simulink model "Kirk_Phase3"  (R2020a)
settings: Solver=FixedStepAuto  StartTime=0.0  StopTime=tsim  FixedStep=baseRate  RelTol=1e-3  EnableMultiTasking=on
values from neighbouring files (symbols this model uses):
  a1 = str2double(environment_file(search_start(1)+length(value)+1:search_start(1)+search_end(1)-2))    [Run_Initializer.m]
  a2 = str2double(environment_file(search_start(1)+length(value)+1:search_start(1)+search_end(1)-2))    [Run_Initializer.m]
  a3 = str2double(environment_file(search_start(1)+length(value)+1:search_start(1)+search_end(1)-2))    [Run_Initializer.m]
  b0 = str2double(environment_file(search_start(1)+length(value)+1:search_start(1)+search_end(1)-2))    [Run_Initializer.m]
  b1 = str2double(environment_file(search_start(1)+length(value)+1:search_start(1)+search_end(1)-2))    [Run_Initializer.m]
  b2 = str2double(environment_file(search_start(1)+length(value)+1:search_start(1)+search_end(1)-2))    [Run_Initializer.m]
  baseRate = 1/20    (= 0.05)    [Run_Initializer.m]
  bring_arm_to_rest_time = 3    [Run_Initializer.m]
  drop_states_BLACK = [ 2.33; 1.2; target_starting_angle]    [Run_Initializer.m]
  drop_states_BLUE = [ xLength/2+0.9; yLength/2+0.5; 0]    [Run_Initializer.m]
  drop_states_RED = [ 1.16; 1.2; 0]    [Run_Initializer.m]
  elbow_max_omega = 30*pi/180    (= 0.523598775598)    [Run_Initializer.m]
  F_thrusters_BLACK = 0.25.*ones(8,1)    [Run_Initializer.m]
  F_thrusters_BLUE = 0.25.*ones(8,1)    [Run_Initializer.m]
  F_thrusters_RED = 0.25.*ones(8,1)    [Run_Initializer.m]
  home_states_BLACK = [ 2.33; 1.2; target_starting_angle]    [Run_Initializer.m]
  home_states_BLUE = [ xLength/2-0.9; yLength/2+0.5; 0]    [Run_Initializer.m]
  home_states_RED = [ 1.16; 1.2; 0]    [Run_Initializer.m]
  I0 = str2double(environment_file(search_start(1)+length(value)+1:search_start(1)+search_end(1)-2))    [Run_Initializer.m]
  I1 = str2double(environment_file(search_start(1)+length(value)+1:search_start(1)+search_end(1)-2))    [Run_Initializer.m]
  I2 = str2double(environment_file(search_start(1)+length(value)+1:search_start(1)+search_end(1)-2))    [Run_Initializer.m]
  I3 = str2double(environment_file(search_start(1)+length(value)+1:search_start(1)+search_end(1)-2))    [Run_Initializer.m]
  init_states_BLACK = [ 2.33; 1.2; target_starting_angle]    [Run_Initializer.m]
  init_states_BLUE = [ xLength/2+0.9; yLength/2+0.5; 0]    [Run_Initializer.m]
  init_states_RED = [ 1.16; 1.2; 0]    [Run_Initializer.m]
  joint_limit_buffer_angle = 0    [Run_Initializer.m]
  Kd_tb = 0.4/5    (= 0.08)    [Run_Initializer.m]
  Kd_tblue = 0.4    [Run_Initializer.m]
  Kd_tr = 0.4    [Run_Initializer.m]
  Kd_xb = 5    [Run_Initializer.m]
  Kd_xblue = 5    [Run_Initializer.m]
  Kd_xr = 5    [Run_Initializer.m]
  Kd_yb = 5    [Run_Initializer.m]
  Kd_yblue = 5    [Run_Initializer.m]
  Kd_yr = 5    [Run_Initializer.m]
  KI_vel_PI = 0    [Run_Initializer.m]
  KI_vel_PI_theta = 0    [Run_Initializer.m]
  Kp_tb = 0.1/5    (= 0.02)    [Run_Initializer.m]
  Kp_tblue = 0.1    [Run_Initializer.m]
  Kp_tr = 0.1    [Run_Initializer.m]
  Kp_vel_PI = 40    [Run_Initializer.m]
  Kp_vel_PI_theta = 0.6    [Run_Initializer.m]
  Kp_xb = 2    [Run_Initializer.m]
  Kp_xblue = 2    [Run_Initializer.m]
  Kp_xr = 2    [Run_Initializer.m]
  Kp_yb = 2    [Run_Initializer.m]
  Kp_yblue = 2    [Run_Initializer.m]
  Kp_yr = 2    [Run_Initializer.m]
  m0 = str2double(environment_file(search_start(1)+length(value)+1:search_start(1)+search_end(1)-2))    [Run_Initializer.m]
  m1 = str2double(environment_file(search_start(1)+length(value)+1:search_start(1)+search_end(1)-2))    [Run_Initializer.m]
  m2 = str2double(environment_file(search_start(1)+length(value)+1:search_start(1)+search_end(1)-2))    [Run_Initializer.m]
  m3 = str2double(environment_file(search_start(1)+length(value)+1:search_start(1)+search_end(1)-2))    [Run_Initializer.m]
  max_body_omega = 15*pi/180    (= 0.261799387799)    [Run_Initializer.m]
  max_x_velocity = 0.1    [Run_Initializer.m]
  max_y_velocity = 0.1    [Run_Initializer.m]
  noise_variance_BLACK = 0    [Run_Initializer.m]
  noise_variance_BLUE = 0    [Run_Initializer.m]
  noise_variance_RED = 0    [Run_Initializer.m]
  Phase0_End = Phase0_Duration    (= 5)    [Run_Initializer.m]
  Phase1_End = Phase0_Duration + Phase1_Duration    (= 10)    [Run_Initializer.m]
  Phase2_End = Phase0_Duration + Phase1_Duration +                                   Phase2_Duration    (= 35)    [Run_Initializer.m]
  Phase3_End = Phase0_Duration + Phase1_Duration +                                   Phase2_Duration + Phase3_Duration    (= 95)    [Run_Initializer.m]
  Phase3_SubPhase1_End = Phase2_End + Phase3_SubPhase1_Duration    (= 35)    [Run_Initializer.m]
  Phase3_SubPhase2_End = Phase2_End + Phase3_SubPhase1_Duration +                                   Phase3_SubPhase2_Duration    (= 35)    [Run_Initializer.m]
  Phase3_SubPhase3_End = Phase2_End + Phase3_SubPhase1_Duration +                                   Phase3_SubPhase2_Duration +                                  Phase3_SubPhase3_Duration    (= 35)    [Run_Initializer.m]
  Phase3_SubPhase4_End = Phase2_End + Phase3_SubPhase1_Duration +                                   Phase3_SubPhase2_Duration +                                  Phase3_SubPhase3_Duration +                                  Phase3_SubPhase4_Duration    [Run_Initializer.m]
  Phase4_End = Phase0_Duration + Phase1_Duration +                                   Phase2_Duration + Phase3_Duration +                                   Phase4_Duration    (= 115)    [Run_Initializer.m]
  Phase5_End = Phase0_Duration + Phase1_Duration +                                   Phase2_Duration + Phase3_Duration +                                   Phase4_Duration + Phase5_Duration    (= 120)    [Run_Initializer.m]
  phi = str2num(erase(environment_file(search_start(1)+length(value)+1:search_start(1)+search_end(1)-2),'np.'))    [Run_Initializer.m]
  serverRate = 1/10    (= 0.1)    [Run_Initializer.m]
  shoulder_max_omega = 30*pi/180    (= 0.523598775598)    [Run_Initializer.m]
  target_angular_velocity = 0.    (= 0)    [Run_Initializer.m]
  thruster_dist2CG_BLACK = [83.42;-52.58;55.94;-60.05;54.08;-53.92;77.06;-55.94]    [Run_Initializer.m]
  thruster_dist2CG_BLUE = [83.42;-52.58;55.94;-60.05;54.08;-53.92;77.06;-55.94]    [Run_Initializer.m]
  thruster_dist2CG_RED = [49.92;-78.08;70.46;-63.54;81.08;-50.42;57.44;-75.96]    [Run_Initializer.m]
  wrist_max_omega = 30*pi/180    (= 0.523598775598)    [Run_Initializer.m]
undefined symbols (not defined in the file or in its folder): DiscIntNeverNeededParam, platformSelection, simMode, WhoAmI
libraries: dspstat3 x18, dspsigops x12, raspberrypiBasiclib x10, MainLibrary x10, embdlinuxlib x8, simulink x8, mspfiltlib x3, dsparch4 x3, dspswit3 x2, sensehatlib x1
(part 12 of 12)

== matlab function Kirk_Phase3/Phase #3: Experiment/Change RED Behavior/Sub-Phase #4/Custom Integral Acceleration Controller1/Sample and Hold Data to Match PhaseSpace (RED)/MATLAB Function ==
  data: TIME input; y output; SERVER input
function y = fcn(TIME, SERVER)

if mod(TIME,SERVER) == 0
    y = 1;
else
    y = 0;
end

== matlab function Kirk_Phase3/Phase #3: Experiment/Change RED Behavior/Sub-Phase #4/Custom Integral Acceleration Controller2/Sample and Hold Data to Match PhaseSpace (RED)/MATLAB Function ==
  data: TIME input; y output; SERVER input
function y = fcn(TIME, SERVER)

if mod(TIME,SERVER) == 0
    y = 1;
else
    y = 0;
end

== matlab function Kirk_Phase3/Phase #3: Experiment/Change BLACK Behavior/Sub-Phase #2 /Hough Control/MATLAB Function2 ==
  data: Oy output; z input; Ox output
function [Oy, Ox]   = C3( z )
%C3 gives the rotation matrix about the z-axis for an angle 'z'
%   z - the angle about the z-axis which you rotate
%   A - the rotation matrix

Ox = [cos(z) sin(z); -sin(z) cos(z)]*[1;0];
Oy = [cos(z) sin(z); -sin(z) cos(z)]*[0;1];
end

== matlab function Kirk_Phase3/Phase #3: Experiment/Change BLACK Behavior/Sub-Phase #2 /Hough Control/MATLAB Function3 ==
  data: z input; Ox output
function Ox    = C3( z )
%C3 gives the rotation matrix about the z-axis for an angle 'z'
%   z - the angle about the z-axis which you rotate
%   A - the rotation matrix

Ox = [cos(z) sin(z); -sin(z) cos(z)]*[1;0];
end

== matlab function Kirk_Phase3/Phase #3: Experiment/Change BLACK Behavior/Sub-Phase #2 /Hough Control/MATLAB Function4 ==
  data: Oy input; e_out output; e_in input
function e_out = fcn(Oy, e_in)

a = sign(Oy'*e_in);
e_out = -a*norm(e_in);

== matlab function Kirk_Phase3/Phase #3: Experiment/Change BLACK Behavior/Sub-Phase #3 /Hough Control/MATLAB Function2 ==
  data: Oy output; z input; Ox output
function [Oy, Ox]   = C3( z )
%C3 gives the rotation matrix about the z-axis for an angle 'z'
%   z - the angle about the z-axis which you rotate
%   A - the rotation matrix

Ox = [cos(z) sin(z); -sin(z) cos(z)]*[1;0];
Oy = [cos(z) sin(z); -sin(z) cos(z)]*[0;1];
end

== matlab function Kirk_Phase3/From Force//Torque to PWM Signal/Change BLUE Behavior/Calculate Thruster ON//OFF/MATLAB Function ==
  data: H output; thruster_dist2CG_BLUE parameter; F_thrusters_BLUE parameter
function H = MakeH(thruster_dist2CG_BLUE,F_thrusters_BLUE)

Vec1 = [ -1
         -1
          0 
          0
          1
          1
          0
          0 ];
      
Vec2 = [  0
          0
          1
          1
          0
          0
         -1
         -1 ];
     
Vec3 = thruster_dist2CG_BLUE./1000;

Mat1 = [Vec1, Vec2, Vec3]';

Mat2 = diag((F_thrusters_BLUE./2));

H    = Mat1*Mat2;

end

== matlab function Kirk_Phase3/Phase #3: Experiment/Change BLACK Behavior/Sub-Phase #3 /Hough Control/MATLAB Function3 ==
  data: z input; Ox output
function Ox    = C3( z )
%C3 gives the rotation matrix about the z-axis for an angle 'z'
%   z - the angle about the z-axis which you rotate
%   A - the rotation matrix

Ox = [cos(z) sin(z); -sin(z) cos(z)]*[1;0];
end

== matlab function Kirk_Phase3/Phase #3: Experiment/Change BLACK Behavior/Sub-Phase #3 /Hough Control/MATLAB Function4 ==
  data: Oy input; e_out output; e_in input
function e_out = fcn(Oy, e_in)

a = sign(Oy'*e_in);
e_out = -a*norm(e_in);

== matlab function Kirk_Phase3/Phase #3: Experiment/Change RED Behavior/Sub-Phase #4/wind down upon capture ==
  data: omega1_in input; omega2_in input; omega3_in input; omega1_out output; is_target_captured input; omega2_out output; omega3_out output; serverRate parameter; bring_arm_to_rest_time parameter; accel_time_ms output
function [omega1_out, omega2_out, omega3_out, accel_time_ms] = are_we_winding_down(omega1_in, omega2_in, omega3_in, is_target_captured, serverRate, bring_arm_to_rest_time)

if is_target_captured
    omega1_out = 0;
    omega2_out = 0;
    omega3_out = 0;
    accel_time_ms = bring_arm_to_rest_time*1000;
else
    omega1_out = omega1_in;
    omega2_out = omega2_in;
    omega3_out = omega3_in;
    accel_time_ms = serverRate*1000;
end

== matlab function Kirk_Phase3/Phase #3: Experiment/Change RED Behavior/Sub-Phase #4/wind down upon_capture2 ==
  data: Fx_in input; Fy_in input; Tz_in input; Fx_out output; is_target_captured input; Fy_out output; Tz_out output
function [Fx_out, Fy_out, Tz_out] = are_we_winding_down(Fx_in, Fy_in, Tz_in, is_target_captured)

if is_target_captured
    Fx_out = 0;
    Fy_out = 0;
    Tz_out = 0;
else
    Fx_out = Fx_in;
    Fy_out = Fy_in;
    Tz_out = Tz_in;
end

== matlab function Kirk_Phase3/Phase #3: Experiment/Change RED Behavior/Sub-Phase #4/calculate_mass_matrix ==
  data: q0_d input; M output; q1_d input; q2_d input; q3_d input; I0 parameter; I1 parameter; I2 parameter; I3 parameter; a1 parameter; a2 parameter; a3 parameter; b0 parameter; b1 parameter; b2 parameter; m0 parameter; m1 parameter; m2 parameter; m3 parameter; phi parameter
function M  = generate_M(q0_d,q1_d,q2_d,q3_d,I0, I1, I2, I3, a1, a2, a3, b0, b1, b2, m0, m1, m2, m3, phi)

t2 = a1+b1;
t3 = a1.*m1;
t4 = m2.*t2;
t5 = m3.*t2;
t6 = q0_d+q1_d;
t7 = cos(t6);
t8 = t3+t4+t5;           
t9 = a2.*m2;
t10 = a2+b2;
t11 = m3.*t10;
t12 = q0_d+q1_d+q2_d;
t13 = cos(t12);
t14 = t9+t11;
t15 = q0_d+q1_d+q2_d+q3_d;
t16 = cos(t15);
t17 = m0+m1+m2+m3;
t18 = b0.*m1;
t19 = b0.*m2;
t20 = b0.*m3;
t21 = t18+t19+t20;
t22 = phi+q0_d;
t23 = sin(t6);
t24 = sin(t12);
t25 = sin(t15);
t26 = a2.*m3;
t27 = b2.*m3;
t28 = t9+t26+t27;
t29 = sin(t22);
t86 = t7.*t8;
t87 = t13.*t14;
t88 = a3.*m3.*t16;
t30 = -t86-t87-t88-t21.*t29;
t31 = cos(t22);
t32 = t21.*t31;
t89 = t8.*t23;
t90 = t14.*t24;
t91 = a3.*m3.*t25;
t33 = t32-t89-t90-t91;
t34 = a1.^2;
t35 = a2.^2;
t36 = b0.^2;
t37 = b1.^2;
t38 = a1.*a2.*m2.*2.0;
t39 = a1.*a2.*m3.*2.0;
t40 = a2.*b1.*m2.*2.0;
t41 = a1.*b2.*m3.*2.0;
t42 = a2.*b1.*m3.*2.0;
t43 = b1.*b2.*m3.*2.0;
t44 = t38+t39+t40+t41+t42+t43;
t45 = cos(q2_d);
t46 = t44.*t45;
t47 = a2.*a3.*m3.*2.0;
t48 = a3.*b2.*m3.*2.0;
t49 = t47+t48;
t50 = cos(q3_d);
t51 = t49.*t50;
t52 = a1.*a3.*m3.*2.0;
t53 = a3.*b1.*m3.*2.0;
t54 = t52+t53;
t55 = q2_d+q3_d;
t56 = cos(t55);
t57 = t54.*t56;
t58 = phi-q1_d;
t59 = sin(t58);
t60 = -phi+q1_d+q2_d;
t61 = sin(t60);
t62 = -phi+q1_d+q2_d+q3_d;
t63 = sin(t62);
t64 = m1.*t34;
t65 = m2.*t34;
t66 = m3.*t34;
t67 = m2.*t35;
t68 = m3.*t35;
t69 = a3.^2;
t70 = m3.*t69;
t71 = m2.*t37;
t72 = m3.*t37;
t73 = b2.^2;
t74 = m3.*t73;
t75 = a1.*b1.*m2.*2.0;
t76 = a1.*b1.*m3.*2.0;
t77 = a2.*b2.*m3.*2.0;
t78 = a2.*b0.*m2;
t79 = a2.*b0.*m3;
t80 = b0.*b2.*m3;
t81 = t78+t79+t80;
t82 = a1.*a3.*m3;
t83 = a3.*b1.*m3;
t84 = t82+t83;
t85 = t56.*t84;
t92 = a1.*b0.*m1;
t93 = a1.*b0.*m2;
t94 = a1.*b0.*m3;
t95 = b0.*b1.*m2;
t96 = b0.*b1.*m3;
t97 = t92+t93+t94+t95+t96;
t98 = t59.*t97;
t112 = t61.*t81;
t113 = a3.*b0.*m3.*t63;
t99 = I1+I2+I3+t46+t51+t57+t64+t65+t66+t67+t68+t70+t71+t72+t74+t75+t76+t77+t98-t112-t113;
t100 = a1.*a2.*m2;
t101 = a1.*a2.*m3;
t102 = a2.*b1.*m2;
t103 = a1.*b2.*m3;
t104 = a2.*b1.*m3;
t105 = b1.*b2.*m3;
t106 = t100+t101+t102+t103+t104+t105;
t107 = t45.*t106;
t108 = a2.*a3.*m3;
t109 = a3.*b2.*m3;
t110 = t108+t109;
t111 = t50.*t110;
t114 = I2+I3+t51+t67+t68+t70+t74+t77+t85+t107;
t115 = I3+t70+t85+t111;
t116 = I3+t70+t111;
M = reshape([t17,0.0,t30,-t86-t87-t88,-t88-t13.*t28,-t88,0.0,t17,t33,-t89-t90-t91,-t91-t24.*t28,-t91,t30,t33,I0+I1+I2+I3+t46+t51+t57+t64+t65+t66+t67+t68+t70+t71+t72+t74+t75+t76+t77+t59.*(a1.*b0.*m1.*2.0+a1.*b0.*m2.*2.0+a1.*b0.*m3.*2.0+b0.*b1.*m2.*2.0+b0.*b1.*m3.*2.0)+m1.*t36+m2.*t36+m3.*t36-t61.*(a2.*b0.*m2.*2.0+a2.*b0.*m3.*2.0+b0.*b2.*m3.*2.0)-a3.*b0.*m3.*t63.*2.0,t99,I2+I3+t51+t67+t68+t70+t74+t77+t85+t107-t112-t113,I3+t70+t85+t111-t113,-t7.*t8-t13.*t14-a3.*m3.*t16,-t8.*t23-t14.*t24-a3.*m3.*t25,t99,I1+I2+I3+t46+t51+t57+t64+t65+t66+t67+t68+t70+t71+t72+t74+t75+t76+t77,t114,t115,-t13.*t28-a3.*m3.*t16,-t24.*t28-a3.*m3.*t25,I2+I3+t51+t67+t68+t70+t74+t77+t85+t107-t61.*t81-a3.*b0.*m3.*t63,t114,I2+I3+t51+t67+t68+t70+t74+t77,t116,-a3.*m3.*t16,-a3.*m3.*t25,I3+t70+t85+t111-a3.*b0.*m3.*t63,t115,t116,I3+t70],[6,6]);

== matlab function Kirk_Phase3/Phase #3: Experiment/Change RED Behavior/Sub-Phase #4/calculate_coriolis_matrix ==
  data: q0_d input; C output; q1_d input; q2_d input; q3_d input; q0_dot_d input; q1_dot_d input; q2_dot_d input; q3_dot_d input; a1 parameter; a2 parameter; a3 parameter; b0 parameter; b1 parameter; b2 parameter; m1 parameter; m2 parameter; m3 parameter; phi parameter
function C  = generate_C(q0_d,q1_d,q2_d,q3_d, q0_dot_d,q1_dot_d,q2_dot_d,q3_dot_d, a1, a2, a3, b0, b1, b2, m1, m2, m3, phi)

t2 = a1+b1;
t3 = a1.*m1;
t4 = m2.*t2;
t5 = m3.*t2;
t6 = t3+t4+t5;
t7 = a2.*m2;
t8 = a2+b2;
t9 = m3.*t8;
t10 = t7+t9;
t11 = pi.*(1.0./2.0);
t12 = q0_dot_d.*t6;
t13 = q1_dot_d.*t6;
t14 = q0_d+q1_d+t11;
t15 = cos(t14);
t16 = t12+t13;
t17 = q0_dot_d.*t10;
t18 = q1_dot_d.*t10;
t19 = q2_dot_d.*t10;
t20 = q0_d+q1_d+q2_d+t11;
t21 = cos(t20);
t22 = t17+t18+t19;
t23 = a3.*m3.*q0_dot_d;
t24 = a3.*m3.*q1_dot_d;
t25 = a3.*m3.*q2_dot_d;
t26 = a3.*m3.*q3_dot_d;
t27 = q0_d+q1_d+q2_d+q3_d+t11;
t28 = cos(t27);
t29 = t23+t24+t25+t26;
t30 = b0.*m1;
t31 = b0.*m2;
t32 = b0.*m3;
t33 = t30+t31+t32;
t34 = phi+q0_d;
t35 = sin(t14);
t36 = sin(t20);
t37 = sin(t27);
t38 = q0_dot_d+q1_dot_d+q2_dot_d+q3_dot_d;
t39 = q0_d+q1_d+q2_d+q3_d;
t40 = a1.*b0.*m1.*q1_dot_d;
t41 = a1.*b0.*m2.*q1_dot_d;
t42 = a1.*b0.*m3.*q1_dot_d;
t43 = b0.*b1.*m2.*q1_dot_d;
t44 = b0.*b1.*m3.*q1_dot_d;
t45 = phi-q1_d;
t46 = cos(t45);
t47 = a2.*b0.*m2.*q1_dot_d;
t48 = a2.*b0.*m2.*q2_dot_d;
t49 = a2.*b0.*m3.*q1_dot_d;
t50 = a2.*b0.*m3.*q2_dot_d;
t51 = b0.*b2.*m3.*q1_dot_d;
t52 = b0.*b2.*m3.*q2_dot_d;
t53 = -phi+q1_d+q2_d;
t54 = cos(t53);
t55 = a3.*b0.*m3.*q1_dot_d;
t56 = a3.*b0.*m3.*q2_dot_d;
t57 = a3.*b0.*m3.*q3_dot_d;
t58 = -phi+q1_d+q2_d+q3_d;
t59 = cos(t58);
t60 = a2.*b1.*m2.*q2_dot_d;
t61 = a1.*b2.*m3.*q2_dot_d;
t62 = a2.*b1.*m3.*q2_dot_d;
t63 = b1.*b2.*m3.*q2_dot_d;
t64 = a1.*a2.*m2.*q2_dot_d;
t65 = a1.*a2.*m3.*q2_dot_d;
t66 = sin(q2_d);
t67 = t60+t61+t62+t63+t64+t65;
t68 = a3.*b2.*m3.*q3_dot_d;
t69 = a2.*a3.*m3.*q3_dot_d;
t70 = sin(q3_d);
t71 = t68+t69;
t72 = a3.*b1.*m3.*q2_dot_d;
t73 = a3.*b1.*m3.*q3_dot_d;
t74 = a1.*a3.*m3.*q2_dot_d;
t75 = a1.*a3.*m3.*q3_dot_d;
t76 = q2_d+q3_d;
t77 = sin(t76);
t78 = t72+t73+t74+t75;
t79 = a2.*b0.*m2.*q0_dot_d;
t80 = a2.*b0.*m3.*q0_dot_d;
t81 = b0.*b2.*m3.*q0_dot_d;
t82 = t47+t48+t49+t50+t51+t52+t79+t80+t81;
t83 = a3.*b0.*m3.*q0_dot_d;
t84 = t55+t56+t57+t83;
t85 = a1.*b0.*m1.*q0_dot_d;
t86 = a1.*b0.*m2.*q0_dot_d;
t87 = a1.*b0.*m3.*q0_dot_d;
t88 = b0.*b1.*m2.*q0_dot_d;
t89 = b0.*b1.*m3.*q0_dot_d;
t90 = a2.*b1.*m2.*q0_dot_d;
t91 = a1.*b2.*m3.*q0_dot_d;
t92 = a2.*b1.*m2.*q1_dot_d;
t93 = a2.*b1.*m3.*q0_dot_d;
t94 = a1.*b2.*m3.*q1_dot_d;
t95 = a2.*b1.*m3.*q1_dot_d;
t96 = b1.*b2.*m3.*q0_dot_d;
t97 = b1.*b2.*m3.*q1_dot_d;
t98 = a1.*a2.*m2.*q0_dot_d;
t99 = a1.*a2.*m2.*q1_dot_d;
t100 = a1.*a2.*m3.*q0_dot_d;
t101 = a1.*a2.*m3.*q1_dot_d;
t102 = t60+t61+t62+t63+t64+t65+t90+t91+t92+t93+t94+t95+t96+t97+t98+t99+t100+t101;
t103 = a3.*b1.*m3.*q0_dot_d;
t104 = a3.*b1.*m3.*q1_dot_d;
t105 = a1.*a3.*m3.*q0_dot_d;
t106 = a1.*a3.*m3.*q1_dot_d;
t107 = t72+t73+t74+t75+t103+t104+t105+t106;
t108 = t79+t80+t81;
t109 = t54.*t108;
t110 = t59.*t83;
t111 = t90+t91+t92+t93+t94+t95+t96+t97+t98+t99+t100+t101;
t112 = t66.*t111;
t113 = t103+t104+t105+t106;
t114 = t77.*t113;
t115 = a2.*q0_dot_d;
t116 = a2.*q1_dot_d;
t117 = a2.*q2_dot_d;
t118 = b2.*q0_dot_d;
t119 = b2.*q1_dot_d;
t120 = b2.*q2_dot_d;
t121 = t115+t116+t117+t118+t119+t120;
t122 = a3.*m3.*t70.*t121;
t123 = a1.*q0_dot_d;
t124 = a1.*q1_dot_d;
t125 = b1.*q0_dot_d;
t126 = b1.*q1_dot_d;
t127 = t123+t124+t125+t126;
t128 = a3.*m3.*t77.*t127;
C = reshape([0.0,0.0,0.0,0.0,0.0,0.0,0.0,0.0,0.0,0.0,0.0,0.0,-t15.*t16-t21.*t22-t28.*t29-q0_dot_d.*t33.*cos(t34),-t16.*t35-t22.*t36-t29.*t37-q0_dot_d.*t33.*sin(t34),-t66.*t67-t70.*t71-t77.*t78-t46.*(t40+t41+t42+t43+t44)-t59.*(t55+t56+t57)-t54.*(t47+t48+t49+t50+t51+t52),t109+t110-t66.*t67-t70.*t71-t77.*t78+t46.*(t85+t86+t87+t88+t89),t109+t110+t112+t114-t70.*t71,t110+t122+t128,-t15.*t16-t21.*t22-t28.*t29,-t16.*t35-t22.*t36-t29.*t37,-t66.*t67-t54.*t82-t70.*t71-t59.*t84-t77.*t78-t46.*(t40+t41+t42+t43+t44+t85+t86+t87+t88+t89),-t66.*t67-t70.*t71-t77.*t78,t112+t114-t70.*t71,t122+t128,-t21.*t22-t28.*t29,-t22.*t36-t29.*t37,-t54.*t82-t70.*t71-t59.*t84-t66.*t102-t77.*t107,-t70.*t71-t66.*t102-t77.*t107,-a3.*m3.*q3_dot_d.*t8.*t70,a3.*m3.*t8.*t70.*(q0_dot_d+q1_dot_d+q2_dot_d),a3.*m3.*t38.*sin(t39),-a3.*m3.*t38.*cos(t39),-a3.*b0.*m3.*t38.*t59-a3.*m3.*t8.*t38.*t70-a3.*m3.*t2.*t38.*t77,-a3.*m3.*t8.*t38.*t70-a3.*m3.*t2.*t38.*t77,-a3.*m3.*t8.*t38.*t70,0.0],[6,6]);

== matlab function Kirk_Phase3/From Force//Torque to PWM Signal/Change BLUE Behavior/Calculate Thruster ON//OFF/MATLAB Function1 ==
  data: H output; thruster_dist2CG_BLUE parameter; F_thrusters_BLUE parameter
function H = MakeH(thruster_dist2CG_BLUE,F_thrusters_BLUE)

Vec1 = [ -1
         -1
          0 
          0
          1
          1
          0
          0 ];
      
Vec2 = [  0
          0
          1
          1
          0
          0
         -1
         -1 ];
     
Vec3 = thruster_dist2CG_BLUE./1000;

Mat1 = [Vec1, Vec2, Vec3]';

Mat2 = diag((F_thrusters_BLUE./2));

H    = Mat1*Mat2;

end

== matlab function Kirk_Phase3/From Force//Torque to PWM Signal/Change RED Behavior/Calculate Thruster ON//OFF/MATLAB Function3 ==
  data: H output; thruster_dist2CG_RED parameter; F_thrusters_RED parameter
function H = MakeH(thruster_dist2CG_RED,F_thrusters_RED)

Vec1 = [ -1
         -1
          0 
          0
          1
          1
          0
          0 ];
      
Vec2 = [  0
          0
          1
          1
          0
          0
         -1
         -1 ];
     
Vec3 = thruster_dist2CG_RED./1000;

Mat1 = [Vec1, Vec2, Vec3]';

Mat2 = diag((F_thrusters_RED./2));

H    = Mat1*Mat2;

end

== matlab function Kirk_Phase3/From Force//Torque to PWM Signal/Change RED Behavior/Calculate Thruster ON//OFF/MATLAB Function4 ==
  data: H output; thruster_dist2CG_RED parameter; F_thrusters_RED parameter; theta_1 input; theta_2 input; theta_3 input; b0 parameter; phi parameter; a1 parameter; b1 parameter; a2 parameter; b2 parameter; a3 parameter; m0 parameter; m1 parameter; m2 parameter; m3 parameter
function H = MakeH(thruster_dist2CG_RED,F_thrusters_RED, theta_1, theta_2, theta_3, b0, phi, a1, b1, a2, b2, a3,m0, m1, m2, m3)

link1_com_x = b0*cos(phi) + a1*cos(pi/2 + theta_1);
link1_com_y = b0*sin(phi) + a1*sin(pi/2 + theta_1);

link2_com_x = link1_com_x + b1*cos(pi/2 + theta_1) + a2*cos(pi/2 + theta_1 + theta_2);
link2_com_y = link1_com_y + b1*sin(pi/2 + theta_1) + a2*sin(pi/2 + theta_1 + theta_2);

link3_com_x = link2_com_x + b2*cos(pi/2 + theta_1 + theta_2) + a3*cos(pi/2 + theta_1 + theta_2 + theta_3);
link3_com_y = link2_com_y + b2*sin(pi/2 + theta_1 + theta_2) + a3*sin(pi/2 + theta_1 + theta_2 + theta_3);

delta_com_due_to_arm_x = (m1*link1_com_x + m2*link2_com_x + m3*link3_com_x)/(m0 + m1 + m2 + m3)*1000; % [mm]
delta_com_due_to_arm_y = (m1*link1_com_y + m2*link2_com_y + m3*link3_com_y)/(m0 + m1 + m2 + m3)*1000; % [mm]

adjusted_thruster_dist2CG_RED = [thruster_dist2CG_RED(1)-delta_com_due_to_arm_y;
                                 thruster_dist2CG_RED(2)-delta_com_due_to_arm_y;
                                 thruster_dist2CG_RED(3)-delta_com_due_to_arm_x;
                                 thruster_dist2CG_RED(4)-delta_com_due_to_arm_x;
                                 thruster_dist2CG_RED(5)+delta_com_due_to_arm_y;
                                 thruster_dist2CG_RED(6)+delta_com_due_to_arm_y;
                                 thruster_dist2CG_RED(7)+delta_com_due_to_arm_x;
                                 thruster_dist2CG_RED(8)+delta_com_due_to_arm_x];
                                 


Vec1 = [ -1
         -1
          0 
          0
          1
          1
          0
          0 ];
      
Vec2 = [  0
          0
          1
          1
          0
          0
         -1
         -1 ];
     
Vec3 = adjusted_thruster_dist2CG_RED./1000;

Mat1 = [Vec1, Vec2, Vec3]';

Mat2 = diag((F_thrusters_RED));

H    = Mat1*Mat2;

end

== matlab function Kirk_Phase3/Phase #3: Experiment/Change RED Behavior/Sub-Phase #4/wind down upon_capture1 ==
  data: Fx_in input; Fy_in input; Tz_in input; Fx_out output; is_target_captured input; Fy_out output; Tz_out output
function [Fx_out, Fy_out, Tz_out] = are_we_winding_down(Fx_in, Fy_in, Tz_in, is_target_captured)

if is_target_captured
    Fx_out = 0;
    Fy_out = 0;
    Tz_out = 0;
else
    Fx_out = Fx_in;
    Fy_out = Fy_in;
    Tz_out = Tz_in;
end

== matlab function Kirk_Phase3/From Force//Torque to PWM Signal/Change BLUE Behavior/Calculate Thruster ON//OFF/MATLAB Function2 ==
  data: ThrustPer_Final output; ThrustPer input
function ThrustPer_Final  = ThrusterSat(ThrustPer)

ValveTime       = 0.007;
TControl        = 0.1;
ThrustPer_Final = zeros(8,1);

if max(ThrustPer) > 1
    ThrustPer_Sat = ThrustPer/max(ThrustPer);
else
    ThrustPer_Sat = ThrustPer;
end

for i = 1:8
    if ThrustPer_Sat(i) > ValveTime/TControl 
        ThrustPer_Final(i) = ThrustPer_Sat(i);
    else
        ThrustPer_Final(i) = 0;
    end
end
   

end

== matlab function Kirk_Phase3/From Force//Torque to PWM Signal/Change BLUE Behavior/Calculate Thruster ON//OFF/Rotate Forces to Inertial/Create Rotation Matrix ==
  data: Rz input; C_Ib output
function C_Ib = RotateFrame(Rz)

C_bI = [  cos(Rz) sin(Rz)
         -sin(Rz) cos(Rz) ];

C_Ib = inv(C_bI);

end
